simulink model "ReadJoystick"  (R2025b)
settings: Solver=FixedStepAuto  StartTime=0.0  StopTime=inf  FixedStep=Ts  RelTol=1e-3
model workspace (MATLAB code in the model file):
  | Ts = 1e-3;
libraries: sl3dlib x1
settings Model: Creator=Asus  LastModifiedBy=Asus
settings OptimizationCC: DefaultParameterBehavior=Inlined  EnhancedBackFolding=on  PassReuseOutputArgsAs=Individual arguments  ZeroExternalMemoryAtStartup=off  ZeroInternalMemoryAtStartup=off  MaxStackSize=64  OptimizeBlockOrder=speed  DifferentSizesBufferReuse=on  OptimizationCustomize=off  EfficientTunableParamExpr=on
settings DebuggingCC: ParameterTunabilityLossMsg=error
settings SFSimCC: MATLABDynamicMemAlloc=off
settings RTWCC: SystemTargetFile=ert.tlc  HardwareBoard=Robot Operating System 2 (ROS 2)  TLCOptions="-aInlineSetEventsForThisBaseRateFcn=TLC_FALSE -aSuppressMultiTaskScheduler=TLC_FALSE  -aRateBasedStepFcn=0"  TemplateMakefile=ert_default_tmf  Toolchain=Colcon Tools  TargetLang=C++  Description=Embedded Coder
settings CodeAppCC: ForceParamTrailComments=on  IgnoreCustomStorageClasses=off  MaxIdLength=95.0  OperatorAnnotations=on  SimulinkDataObjDesc=on  SFDataObjDesc=on  InsertBlockDesc=on
settings ERTTargetCC: RootIOFormat=Structure reference  CodeInterfacePackaging=C++ class

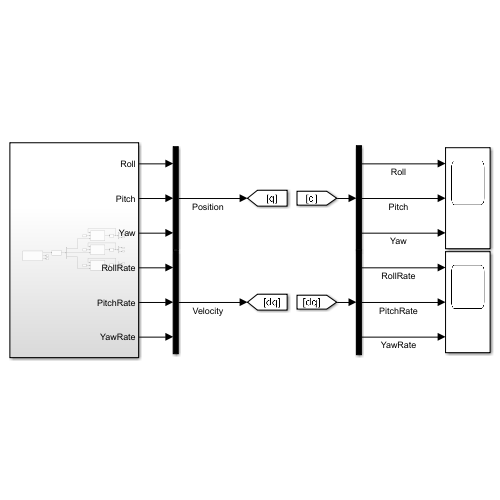
[thumbnail: Simulink's stored preview of the top-level diagram]
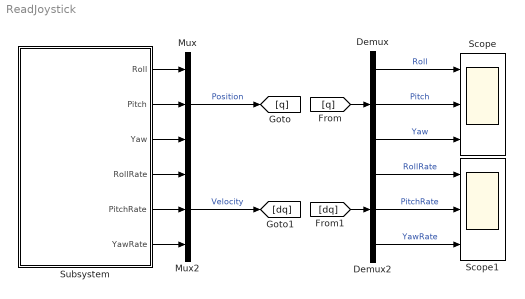
== system ReadJoystick ==
  Demux : Demux  Outputs=3
  Demux2 : Demux  Outputs=3
  Mux : Mux  Inputs=3
  Mux2 : Mux  Inputs=3
  Scope : Scope  NumInputPorts=3
      settings: ActiveDisplayYMinimum=-0.34633574718669058  ActiveDisplayYMaximum=0.34393074192782541
  Scope1 : Scope  NumInputPorts=3
      settings: ActiveDisplayYMinimum=-2.5156139726495823  ActiveDisplayYMaximum=2.3658078903480848
  Subsystem : Subsystem
  wires:
  Subsystem/1(Roll) -> Mux/1
  Mux/1 -> [q]  "Position"
  Subsystem/2(Pitch) -> Mux/2
  Subsystem/3(Yaw) -> Mux/3
  Mux2/1 -> [dq]  "Velocity"
  Subsystem/4(RollRate) -> Mux2/1
  Subsystem/5(PitchRate) -> Mux2/2
  Subsystem/6(YawRate) -> Mux2/3
  [dq] -> Demux2/1
  [q] -> Demux/1
  Demux/2 -> Scope/2  "Pitch"
  Demux/1 -> Scope/1  "Roll"
  Demux/3 -> Scope/3  "Yaw"
  Demux2/1 -> Scope1/1  "RollRate"
  Demux2/2 -> Scope1/2  "PitchRate"
  Demux2/3 -> Scope1/3  "YawRate"

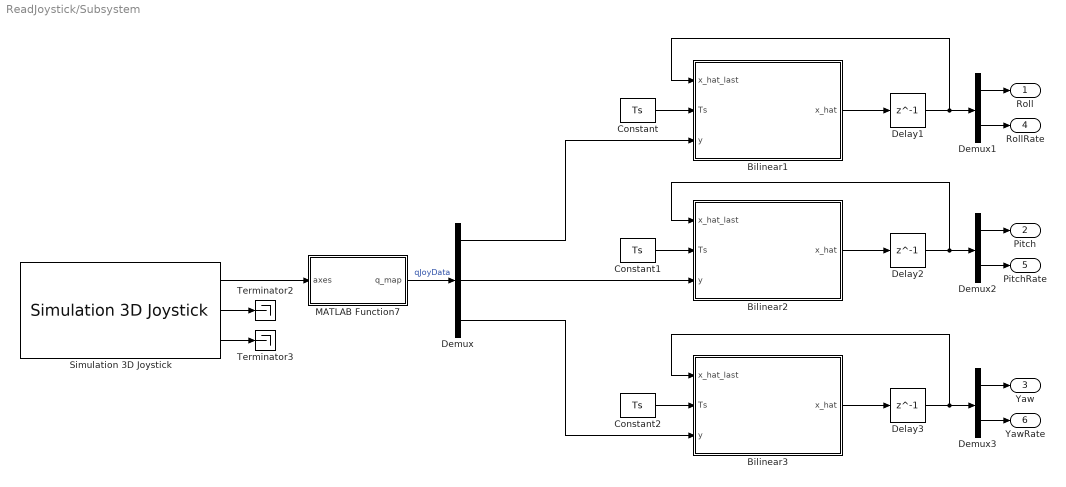
== system ReadJoystick/Subsystem ==
  Bilinear1 : MATLAB Function  TreatAsAtomicUnit=on
  Bilinear2 : MATLAB Function  TreatAsAtomicUnit=on
  Bilinear3 : MATLAB Function  TreatAsAtomicUnit=on
  Constant : Constant  Value=Ts
  Constant1 : Constant  Value=Ts
  Constant2 : Constant  Value=Ts
  Delay1 : Delay  DelayLength=1  InitialCondition=[0; 0]
  Delay2 : Delay  DelayLength=1  InitialCondition=[0; 0]
  Delay3 : Delay  DelayLength=1  InitialCondition=[0; 0]
  Demux : Demux  Outputs=3
  Demux1 : Demux  Outputs=2
  Demux2 : Demux  Outputs=2
  Demux3 : Demux  Outputs=2
  MATLAB Function7 : MATLAB Function  TreatAsAtomicUnit=on
  Simulation 3D Joystick : sl3dlib/Simulation 3D/Hardware Interface/Simulation 3D Joystick  joyid=1  adjustports=on  forcefeed=off
  Terminator2 : Terminator
  Terminator3 : Terminator
  Roll : Outport
  Pitch : Outport  Port=2
  Yaw : Outport  Port=3
  RollRate : Outport  Port=4
  PitchRate : Outport  Port=5
  YawRate : Outport  Port=6
  wires:
  Delay1/1 -> Bilinear1/1(x_hat_last), Demux1/1
  Bilinear2/1(x_hat) -> Delay2/1
  Bilinear1/1(x_hat) -> Delay1/1
  Bilinear3/1(x_hat) -> Delay3/1
  Delay2/1 -> Demux2/1, Bilinear2/1(x_hat_last)
  Delay3/1 -> Demux3/1, Bilinear3/1(x_hat_last)
  Demux/1 -> Bilinear1/3(y)
  Demux/2 -> Bilinear2/3(y)
  Demux/3 -> Bilinear3/3(y)
  Demux1/1 -> Roll/1
  Demux1/2 -> RollRate/1
  Demux2/2 -> PitchRate/1
  Demux2/1 -> Pitch/1
  Demux3/2 -> YawRate/1
  Demux3/1 -> Yaw/1
  Simulation 3D Joystick/1 -> MATLAB Function7/1(axes)
  Simulation 3D Joystick/2 -> Terminator2/1
  Simulation 3D Joystick/3 -> Terminator3/1
  MATLAB Function7/1(q_map) -> Demux/1  "qJoyData"
  Constant/1 -> Bilinear1/2(Ts)
  Constant1/1 -> Bilinear2/2(Ts)
  Constant2/1 -> Bilinear3/2(Ts)

== matlab function ReadJoystick/Subsystem/MATLAB Function7 ==
  data: axes input; q_map output
function q_map = fcn(axes)

    q_map = zeros(3, 1);
    scales = [0.25, -0.5, -1.0];
    q_map(1) = axes(1) * scales(1);
    q_map(2) = axes(2) * scales(2);
    q_map(3) = axes(3) * scales(3);

end

== matlab function ReadJoystick/Subsystem/Bilinear1 ==
  data: x_hat_last input; Ts input; y input; x_hat output
function x_hat = Bilinear(x_hat_last, Ts, y)

    % continuous time system model
    A = [0, 1; 0, 0];
    C = [1, 0];

    % design params
    alpha = 0.1;
    beta  = [6, 5]';
    H     = [beta(1)/alpha, beta(2)/alpha^2]';

    % discrete time system
    Ad = (eye(2) - Ts/2*A) \ (eye(2) + Ts/2*A);
    Hd = Ts * ((eye(2) - Ts/2*A) \ H);

    % observer model
    x_hat = Ad * x_hat_last + Hd * (y - C * x_hat_last);

end

== matlab function ReadJoystick/Subsystem/Bilinear2 ==
  data: x_hat_last input; Ts input; y input; x_hat output
function x_hat = Bilinear(x_hat_last, Ts, y)

    % continuous time system model
    A = [0, 1; 0, 0];
    C = [1, 0];

    % design params
    alpha = 0.1;
    beta  = [6, 5]';
    H     = [beta(1)/alpha, beta(2)/alpha^2]';

    % discrete time system
    Ad = (eye(2) - Ts/2*A) \ (eye(2) + Ts/2*A);
    Hd = Ts * ((eye(2) - Ts/2*A) \ H);

    % observer model
    x_hat = Ad * x_hat_last + Hd * (y - C * x_hat_last);

end

== matlab function ReadJoystick/Subsystem/Bilinear3 ==
  data: x_hat_last input; Ts input; y input; x_hat output
function x_hat = Bilinear(x_hat_last, Ts, y)

    % continuous time system model
    A = [0, 1; 0, 0];
    C = [1, 0];

    % design params
    alpha = 0.1;
    beta  = [6, 5]';
    H     = [beta(1)/alpha, beta(2)/alpha^2]';

    % discrete time system
    Ad = (eye(2) - Ts/2*A) \ (eye(2) + Ts/2*A);
    Hd = Ts * ((eye(2) - Ts/2*A) \ H);

    % observer model
    x_hat = Ad * x_hat_last + Hd * (y - C * x_hat_last);

end
